simulink model "Approx_control"  (R2021b)
settings: Solver=VariableStepAuto  StartTime=0.0  StopTime=10.0  RelTol=1e-3
undefined symbols (not defined in the file or in its folder): A, B, C
libraries: cstblocks x4
settings Model: Creator=pierg  LastModifiedBy=pierg

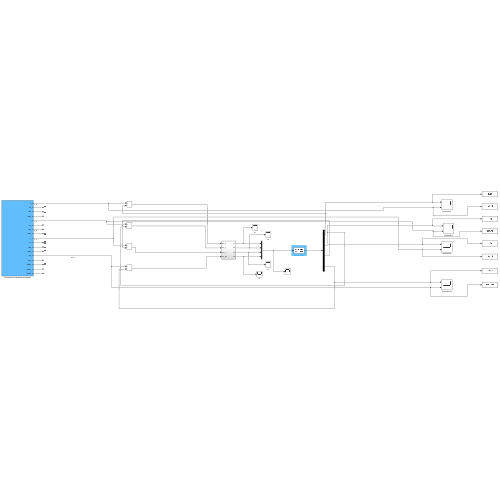
[thumbnail: Simulink's stored preview of the top-level diagram]
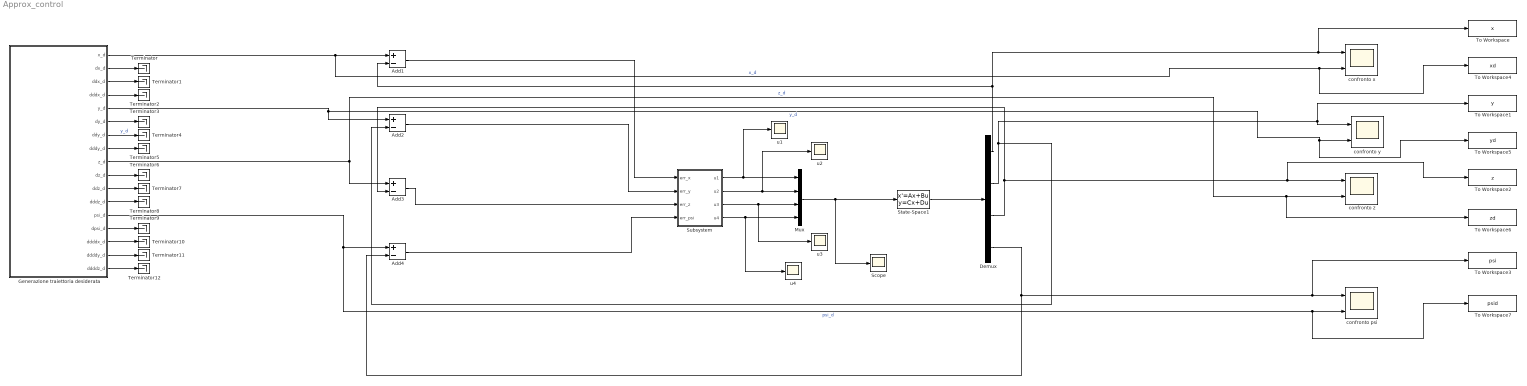
== system Approx_control ==
  Add{1..4} (4 alike) : Sum  Inputs=+-
  Demux : Demux
  Generazione traiettoria desiderata : Subsystem
  Mux : Mux
  Scope : Scope
  State-Space1 : StateSpace  A=A  B=B  C=C  D=zeros(4,4)  InitialCondition=[5 5 10 0 0 0 0 0 pi/4 0 0 0]'  ParameterTunability=Unconstrained
  Subsystem : Subsystem
  Terminator{,1..12} (13 alike) : Terminator
  To Workspace : ToWorkspace  VariableName=x  SaveFormat=Structure  SampleTime=-1
  To Workspace1 : ToWorkspace  VariableName=y  SaveFormat=Structure  SampleTime=-1
  To Workspace2 : ToWorkspace  VariableName=z  SaveFormat=Structure  SampleTime=-1
  To Workspace3 : ToWorkspace  VariableName=psi  SaveFormat=Structure  SampleTime=-1
  To Workspace4 : ToWorkspace  VariableName=xd  SaveFormat=Structure  SampleTime=-1
  To Workspace5 : ToWorkspace  VariableName=yd  SaveFormat=Structure  SampleTime=-1
  To Workspace6 : ToWorkspace  VariableName=zd  SaveFormat=Structure  SampleTime=-1
  To Workspace7 : ToWorkspace  VariableName=psid  SaveFormat=Structure  SampleTime=-1
  confronto psi : Scope  NumInputPorts=2
  confronto x : Scope  NumInputPorts=2
  confronto y : Scope  NumInputPorts=2
  confronto z : Scope  NumInputPorts=2
  u{1..4} (4 alike) : Scope
  wires:
  State-Space1/1 -> Demux/1
  Mux/1 -> State-Space1/1, Scope/1
  Generazione traiettoria desiderata/13(psi_d) -> To Workspace7/1, confronto psi/2, Add4/1  "psi_d"
  Generazione traiettoria desiderata/1(x_d) -> To Workspace4/1, confronto x/2, Add1/1  "x_d"
  Demux/1 -> To Workspace/1, confronto x/1, Add1/2
  Generazione traiettoria desiderata/5(y_d) -> Add2/1, To Workspace5/1, confronto y/2  "y_d"
  Demux/2 -> Add2/2, To Workspace1/1, confronto y/1
  Generazione traiettoria desiderata/9(z_d) -> Add3/1, To Workspace6/1, confronto z/2  "z_d"
  Demux/3 -> Add3/2, To Workspace2/1, confronto z/1
  Subsystem/2(u2) -> u2/1, Mux/2
  Subsystem/4(u4) -> u4/1, Mux/4
  Add1/1 -> Subsystem/1(err_x)
  Add2/1 -> Subsystem/2(err_y)
  Add3/1 -> Subsystem/3(err_z)
  Add4/1 -> Subsystem/4(err_psi)
  Demux/4 -> Add4/2, To Workspace3/1, confronto psi/1
  Subsystem/1(u1) -> u1/1, Mux/1
  Subsystem/3(u3) -> u3/1, Mux/3
  Generazione traiettoria desiderata/2(dx_d) -> Terminator/1
  Generazione traiettoria desiderata/3(ddx_d) -> Terminator1/1
  Generazione traiettoria desiderata/4(dddx_d) -> Terminator2/1
  Generazione traiettoria desiderata/6(dy_d) -> Terminator3/1
  Generazione traiettoria desiderata/7(ddy_d) -> Terminator4/1  "y_d"
  Generazione traiettoria desiderata/8(dddy_d) -> Terminator5/1
  Generazione traiettoria desiderata/10(dz_d) -> Terminator6/1
  Generazione traiettoria desiderata/11(ddz_d) -> Terminator7/1
  Generazione traiettoria desiderata/12(dddz_d) -> Terminator8/1
  Generazione traiettoria desiderata/14(dpsi_d) -> Terminator9/1
  Generazione traiettoria desiderata/15(ddddx_d) -> Terminator10/1
  Generazione traiettoria desiderata/16(ddddy_d) -> Terminator11/1
  Generazione traiettoria desiderata/17(ddddz_d) -> Terminator12/1

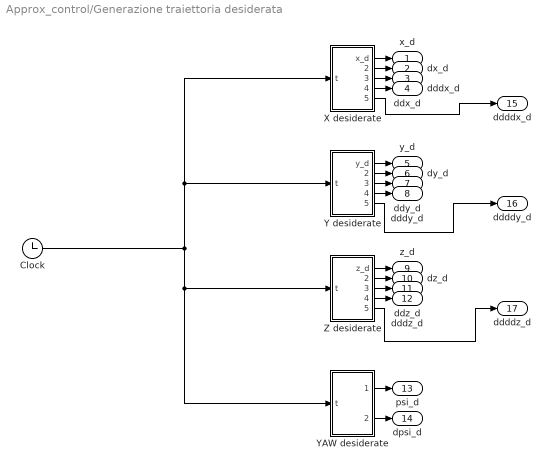
== system Approx_control/Generazione traiettoria desiderata ==
  Clock : Clock
  X desiderate : Subsystem
  Y desiderate : Subsystem
  YAW desiderate : Subsystem
  Z desiderate : Subsystem
  x_d : Outport
  dx_d : Outport  Port=2
  ddx_d : Outport  Port=3
  dddx_d : Outport  Port=4
  y_d : Outport  Port=5
  dy_d : Outport  Port=6
  ddy_d : Outport  Port=7
  dddy_d : Outport  Port=8
  z_d : Outport  Port=9
  dz_d : Outport  Port=10
  ddz_d : Outport  Port=11
  dddz_d : Outport  Port=12
  psi_d : Outport  Port=13
  dpsi_d : Outport  Port=14
  ddddx_d : Outport  Port=15
  ddddy_d : Outport  Port=16
  ddddz_d : Outport  Port=17
  wires:
  Y desiderate/1(y_d) -> y_d/1
  Y desiderate/2(dy_d) -> dy_d/1
  X desiderate/5(ddddx_d) -> ddddx_d/1
  X desiderate/3(ddx_d) -> ddx_d/1
  YAW desiderate/2(dpsi_d) -> dpsi_d/1
  Z desiderate/1(z_d) -> z_d/1
  Z desiderate/4(dddz_d) -> dddz_d/1
  X desiderate/2(dx_d) -> dx_d/1
  Y desiderate/4(dddy_d) -> dddy_d/1
  X desiderate/4(dddx_d) -> dddx_d/1
  Y desiderate/3(ddy_d) -> ddy_d/1
  X desiderate/1(x_d) -> x_d/1
  Z desiderate/5(ddddz_d) -> ddddz_d/1
  Z desiderate/2(dz_d) -> dz_d/1
  YAW desiderate/1(psi_d) -> psi_d/1
  Z desiderate/3(ddz_d) -> ddz_d/1
  Y desiderate/5(ddddy_d) -> ddddy_d/1
  Clock/1 -> YAW desiderate/1(t), Z desiderate/1(t), X desiderate/1(t), Y desiderate/1(t)

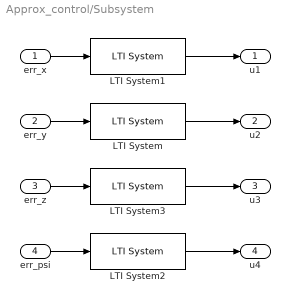
== system Approx_control/Subsystem ==
  err_x : Inport
  err_y : Inport  Port=2
  err_z : Inport  Port=3
  err_psi : Inport  Port=4
  LTI System : cstblocks/LTI System  sys=C2  IC=[]
  LTI System1 : cstblocks/LTI System  sys=C1  IC=[]
  LTI System2 : cstblocks/LTI System  sys=C4  IC=[]
  LTI System3 : cstblocks/LTI System  sys=C3  IC=[]
  u1 : Outport  VectorParamsAs1DForOutWhenUnconnected=off
  u2 : Outport  Port=2  VectorParamsAs1DForOutWhenUnconnected=off
  u3 : Outport  Port=3  VectorParamsAs1DForOutWhenUnconnected=off
  u4 : Outport  Port=4  VectorParamsAs1DForOutWhenUnconnected=off
  wires:
  err_x/1 -> LTI System1/1
  LTI System/1 -> u2/1
  LTI System1/1 -> u1/1
  err_y/1 -> LTI System/1
  err_psi/1 -> LTI System2/1
  LTI System3/1 -> u3/1
  LTI System2/1 -> u4/1
  err_z/1 -> LTI System3/1

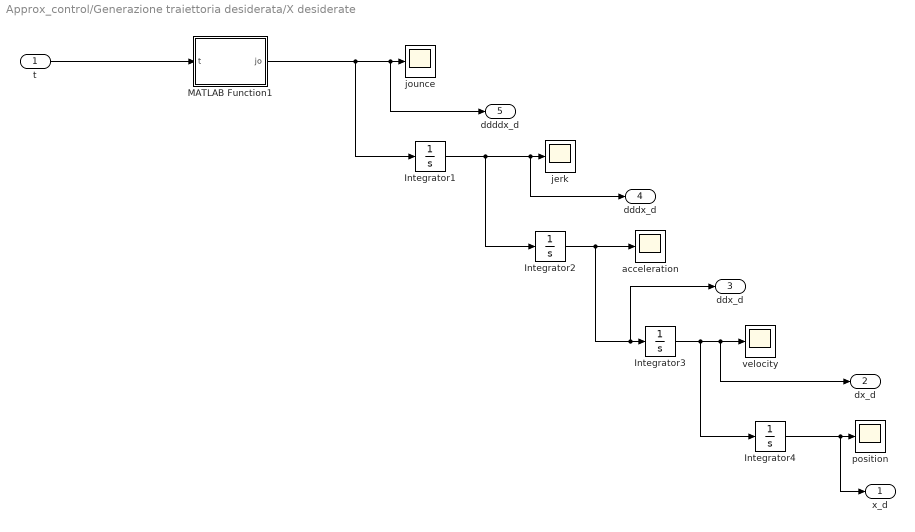
== system Approx_control/Generazione traiettoria desiderata/X desiderate ==
  t : Inport
  Integrator1 : Integrator
  Integrator2 : Integrator
  Integrator3 : Integrator
  Integrator4 : Integrator  InitialCondition=10
  MATLAB Function1 : MATLAB Function  TreatAsAtomicUnit=on
  acceleration : Scope
  jerk : Scope
  jounce : Scope
  position : Scope
  velocity : Scope
  x_d : Outport
  dx_d : Outport  Port=2
  ddx_d : Outport  Port=3
  dddx_d : Outport  Port=4
  ddddx_d : Outport  Port=5
  wires:
  MATLAB Function1/1(jo) -> Integrator1/1, ddddx_d/1, jounce/1
  Integrator4/1 -> x_d/1, position/1
  Integrator3/1 -> Integrator4/1, dx_d/1, velocity/1
  Integrator2/1 -> ddx_d/1, Integrator3/1, acceleration/1
  Integrator1/1 -> Integrator2/1, dddx_d/1, jerk/1
  t/1 -> MATLAB Function1/1(t)

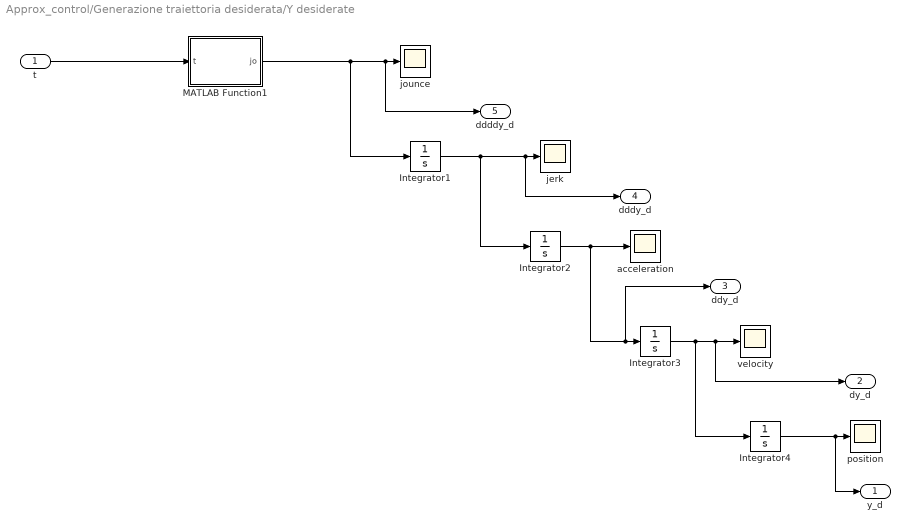
== system Approx_control/Generazione traiettoria desiderata/Y desiderate ==
  t : Inport
  Integrator1 : Integrator
  Integrator2 : Integrator
  Integrator3 : Integrator
  Integrator4 : Integrator  InitialCondition=5
  MATLAB Function1 : MATLAB Function  TreatAsAtomicUnit=on
  acceleration : Scope
  jerk : Scope
  jounce : Scope
  position : Scope
  velocity : Scope
  y_d : Outport
  dy_d : Outport  Port=2
  ddy_d : Outport  Port=3
  dddy_d : Outport  Port=4
  ddddy_d : Outport  Port=5
  wires:
  t/1 -> MATLAB Function1/1(t)
  Integrator1/1 -> jerk/1, dddy_d/1, Integrator2/1
  Integrator2/1 -> acceleration/1, Integrator3/1, ddy_d/1
  Integrator3/1 -> velocity/1, dy_d/1, Integrator4/1
  Integrator4/1 -> position/1, y_d/1
  MATLAB Function1/1(jo) -> jounce/1, ddddy_d/1, Integrator1/1

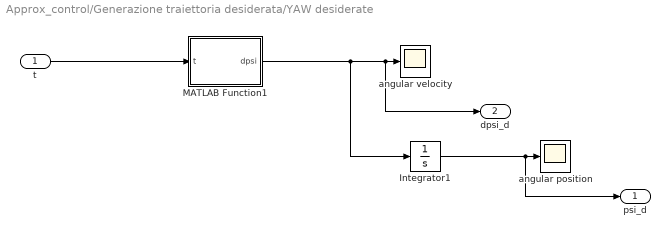
== system Approx_control/Generazione traiettoria desiderata/YAW desiderate ==
  t : Inport
  Integrator1 : Integrator
  MATLAB Function1 : MATLAB Function  TreatAsAtomicUnit=on
  angular position : Scope
  angular velocity : Scope
  psi_d : Outport
  dpsi_d : Outport  Port=2
  wires:
  t/1 -> MATLAB Function1/1(t)
  Integrator1/1 -> angular position/1, psi_d/1
  MATLAB Function1/1(dpsi) -> angular velocity/1, dpsi_d/1, Integrator1/1

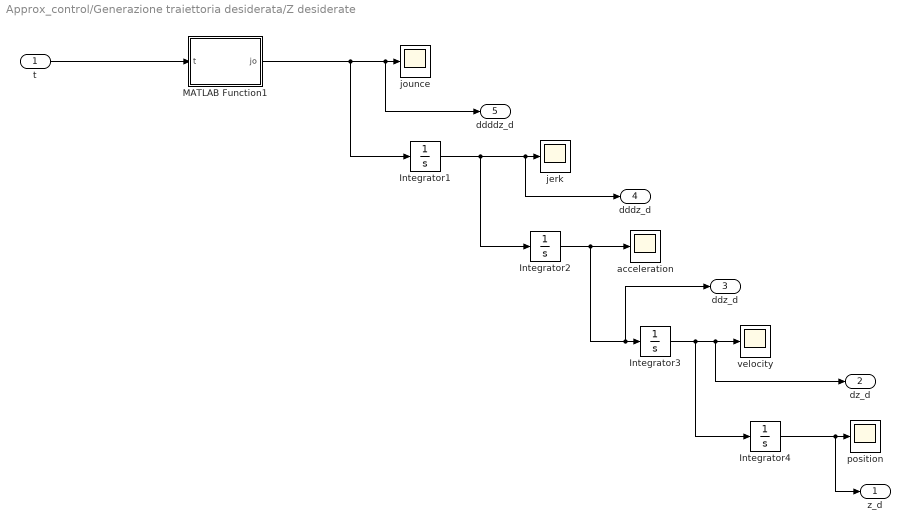
== system Approx_control/Generazione traiettoria desiderata/Z desiderate ==
  t : Inport
  Integrator{1..4} (4 alike) : Integrator
  MATLAB Function1 : MATLAB Function  TreatAsAtomicUnit=on
  acceleration : Scope
  jerk : Scope
  jounce : Scope
  position : Scope
  velocity : Scope
  z_d : Outport
  dz_d : Outport  Port=2
  ddz_d : Outport  Port=3
  dddz_d : Outport  Port=4
  ddddz_d : Outport  Port=5
  wires:
  MATLAB Function1/1(jo) -> Integrator1/1, ddddz_d/1, jounce/1
  Integrator4/1 -> z_d/1, position/1
  Integrator3/1 -> Integrator4/1, dz_d/1, velocity/1
  Integrator2/1 -> ddz_d/1, Integrator3/1, acceleration/1
  Integrator1/1 -> Integrator2/1, dddz_d/1, jerk/1
  t/1 -> MATLAB Function1/1(t)

== matlab function Approx_control/Generazione traiettoria desiderata/Y desiderate/MATLAB Function1 ==
  data: t input; jo output
function jo = jounce(t)
% % Parametri
% a = 1/10;
% b = 1;
% c = 1;
% 
% % Accelerating part
% if t < b
%     j = a * sin(pi*t/b);
% elseif t >= b && t <= 3*b
%     j = -a * sin(pi*t/(2*b)-pi/2);
% elseif t > 3*b && t <= 4*b
%     j = a * sin(pi*t/b-3*pi);
% elseif t > 4*b && t <= 4*b+c
%     j = 0;
% % Decelerating part
% elseif t > 4*b+c && t <= 5*b+c
%     j = a * sin(pi*t/b);
% elseif t > 5*b+c && t <= 7*b+c
%     j = a * sin(0.5*pi*t/(b)+pi);
% elseif t > 7*b+c && t <= 8*b+c
%     j = a * sin(pi*t/b-3*pi);
% else
%     j = 0;
% end

jo = 0;

== matlab function Approx_control/Generazione traiettoria desiderata/Z desiderate/MATLAB Function1 ==
  data: t input; jo output
function jo = jounce(t)
% Parametri
a = 1;
b = 1;
c = 1;

% Accelerating part
if t < b
    j = a * sin(pi*t/b);
elseif t >= b && t <= 3*b
    j = -a * sin(pi*t/(2*b)-pi/2);
elseif t > 3*b && t <= 4*b
    j = a * sin(pi*t/b-3*pi);
elseif t > 4*b && t <= 4*b+c
    j = 0;
% Decelerating part
elseif t > 4*b+c && t <= 5*b+c
    j = a * sin(pi*t/b);
elseif t > 5*b+c && t <= 7*b+c
    j = a * sin(0.5*pi*t/(b)+pi);
elseif t > 7*b+c && t <= 8*b+c
    j = a * sin(pi*t/b-3*pi);
else
    j = 0;
end

jo = j;

== matlab function Approx_control/Generazione traiettoria desiderata/YAW desiderate/MATLAB Function1 ==
  data: t input; dpsi output
function dpsi = ang_vel(t)
% % Parametri
% a = 1/3;
% b = 2;
% c =2;
% 
% % Accelerating part
% if t < b
%     j = a * sin(pi*t/b);
% elseif t >= b && t <= 3*b
%     j = -a * sin(pi*t/(2*b)-pi/2);
% elseif t > 3*b && t <= 4*b
%     j = a * sin(pi*t/b-3*pi);
% elseif t > 4*b && t <= 4*b+c
%     j = 0;
% % Decelerating part
% elseif t > 4*b+c && t <= 5*b+c
%     j = a * sin(pi*t/b);
% elseif t > 5*b+c && t <= 7*b+c
%     j = a * sin(0.5*pi*t/(b)+pi);
% elseif t > 7*b+c && t <= 8*b+c
%     j = a * sin(pi*t/b-3*pi);
% else
%     j = 0;
% end

dpsi = 0*t;

== matlab function Approx_control/Generazione traiettoria desiderata/X desiderate/MATLAB Function1 ==
  data: t input; jo output
function jo = jounce(t)
% % Parametri
% a = 1;
% b = 1;
% c = 1;
% 
% % Accelerating part
% if t < b
%     j = a * sin(pi*t/b);
% elseif t >= b && t <= 3*b
%     j = -a * sin(pi*t/(2*b)-pi/2);
% elseif t > 3*b && t <= 4*b
%     j = a * sin(pi*t/b-3*pi);
% elseif t > 4*b && t <= 4*b+c
%     j = 0;
% % Decelerating part
% elseif t > 4*b+c && t <= 5*b+c
%     j = a * sin(pi*t/b);
% elseif t > 5*b+c && t <= 7*b+c
%     j = a * sin(0.5*pi*t/(b)+pi);
% elseif t > 7*b+c && t <= 8*b+c
%     j = a * sin(pi*t/b-3*pi);
% else
%     j = 0;
% end

jo = 0;
